simulink model "BlokSchema3"  (R2023a)
settings: Solver=VariableStepAuto  StartTime=0.0  StopTime=5000  RelTol=1e-5
undefined symbols (not defined in the file): citatel, Delay, menovatel, p01, p02, p03, p11, p12, p13, q00, q01, q02, q03, q10, q11, q12, q13, T
settings Model: PacingRate=100  Creator=domin  LastModifiedBy=domin

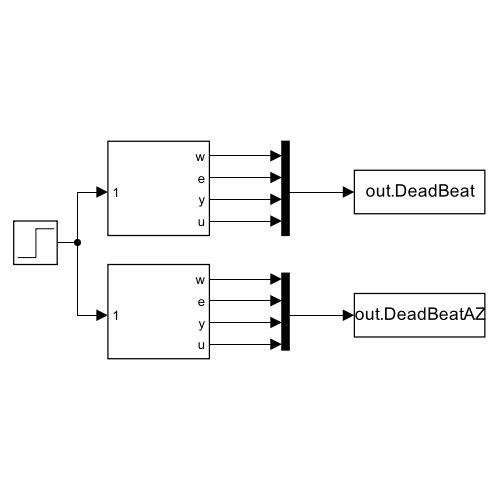
[thumbnail: Simulink's stored preview of the top-level diagram]
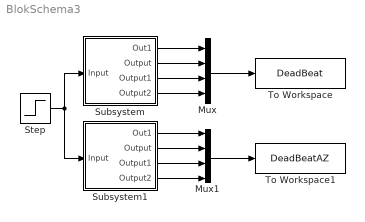
== system BlokSchema3 ==
  Mux : Mux
  Mux1 : Mux
  Step : Step  Time=0  Before=1  SampleTime=0
  Subsystem : Subsystem
  Subsystem1 : Subsystem
  To Workspace : ToWorkspace  VariableName=DeadBeat  SaveFormat=Timeseries  SampleTime=-1
  To Workspace1 : ToWorkspace  VariableName=DeadBeatAZ  SampleTime=-1
  wires:
  Step/1 -> Subsystem/1(Input), Subsystem1/1(Input)
  Subsystem/1(Out1) -> Mux/1
  Subsystem/2(Output) -> Mux/2
  Subsystem/3(Output1) -> Mux/3
  Subsystem/4(Output2) -> Mux/4
  Mux/1 -> To Workspace/1
  Mux1/1 -> To Workspace1/1
  Subsystem1/1(Out1) -> Mux1/1
  Subsystem1/2(Output) -> Mux1/2
  Subsystem1/3(Output1) -> Mux1/3
  Subsystem1/4(Output2) -> Mux1/4

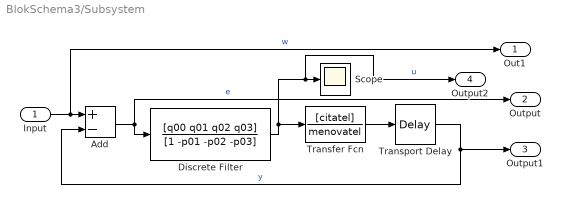
== system BlokSchema3/Subsystem ==
  Input : Inport
  Add : Sum  Inputs=+-
  Discrete Filter : DiscreteFilter  Numerator=[q00 q01 q02 q03]  Denominator=[1 -p01 -p02 -p03]  SampleTime=T
  Scope : Scope
  Transfer Fcn : TransferFcn  Numerator=[citatel]  Denominator=menovatel
  Transport Delay : TransportDelay  DelayTime=Delay
  Out1 : Outport
  Output : Outport  Port=2
  Output1 : Outport  Port=3
  Output2 : Outport  Port=4
  wires:
  Add/1 -> Output/1, Discrete Filter/1  "e"
  Input/1 -> Out1/1, Add/1  "w"
  Transfer Fcn/1 -> Transport Delay/1
  Discrete Filter/1 -> Transfer Fcn/1, Output2/1, Scope/1  "u"
  Transport Delay/1 -> Output1/1, Add/2  "y"

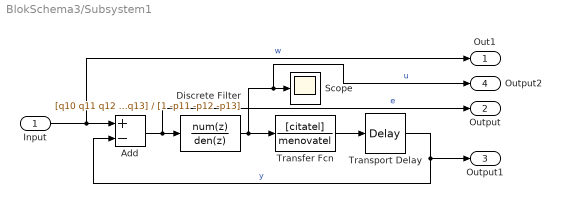
== system BlokSchema3/Subsystem1 ==
  Input : Inport
  Add : Sum  Inputs=+-
  Discrete Filter : DiscreteFilter  Numerator=[q10 q11 q12 q13]  Denominator=[1 -p11 -p12 -p13]  SampleTime=T
  Scope : Scope
  Transfer Fcn : TransferFcn  Numerator=[citatel]  Denominator=menovatel
  Transport Delay : TransportDelay  DelayTime=Delay
  Out1 : Outport
  Output : Outport  Port=2
  Output1 : Outport  Port=3
  Output2 : Outport  Port=4
  wires:
  Add/1 -> Discrete Filter/1, Output/1  "e"
  Input/1 -> Out1/1, Add/1  "w"
  Transfer Fcn/1 -> Transport Delay/1
  Discrete Filter/1 -> Transfer Fcn/1, Output2/1, Scope/1  "u"
  Transport Delay/1 -> Output1/1, Add/2  "y"
